simulink model "Cristian_estimacion_planta_simul"  (R2018a)
settings: Solver=VariableStepAuto  StartTime=0.0  StopTime=250  RelTol=1e-3
undefined symbols (not defined in the file or in its folder): dQ, nQ
libraries: SignalEditorBlockLib x1
settings Model: Creator=quich  LastModifiedBy=quich

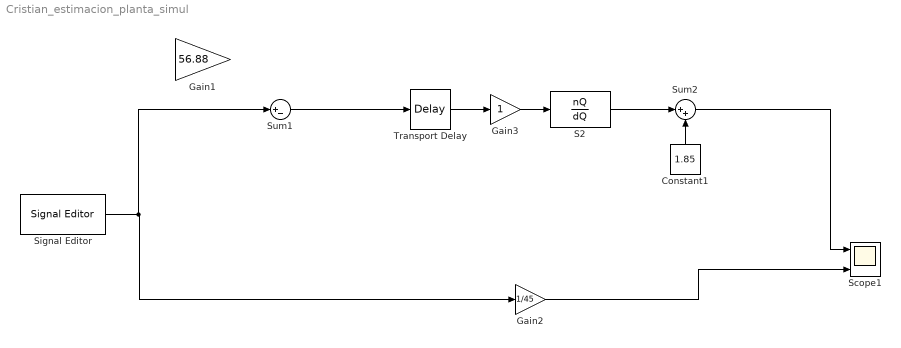
== system Cristian_estimacion_planta_simul ==
  Constant1 : Constant  Value=1.85  SampleTime=0.055
  Gain1 : Gain  Gain=56.88
  Gain2 : Gain  Gain=1/45
  Gain3 : Gain
  S2 : TransferFcn  Numerator=nQ  Denominator=dQ
  Scope1 : Scope  NumInputPorts=3
  Signal Editor : SignalEditorBlockLib/Signal Editor  FileName=Cris_P6.mat  ActiveScenario=Scenario  ActiveSignal=Signal  IsBus=off  OutputBusObjectStr=Bus: BusObject  SampleTime=0  Interpolate=off  ZeroCross=off  OutputAfterFinalValue=Setting to zero  Unit=inherit
  Sum1 : Sum  Inputs=|+-
  Sum2 : Sum  Inputs=|++
  Transport Delay : TransportDelay  DelayTime=1.2
  wires:
  Gain3/1 -> S2/1
  Transport Delay/1 -> Gain3/1
  Sum2/1 -> Scope1/1
  Signal Editor/1 -> Sum1/1, Gain2/1
  Constant1/1 -> Sum2/2
  S2/1 -> Sum2/1
  Sum1/1 -> Transport Delay/1
  Gain2/1 -> Scope1/3
